simulink model "V2G"  (R2024a)
settings: Solver=ode23tb  StartTime=0.0  StopTime=0.3  MaxStep=1e-6  RelTol=1e-3  EnableMultiTasking=on
undefined symbols (not defined in the file): DiscIntNeverNeededParam, Ion, Lithium
libraries: powerlib_extras x6, spsControlledVoltageSourceLib x5, spsSeriesRLCBranchLib x3, simulink x3, spsCurrentMeasurementLib x3, spsACVoltageSourceLib x3, spsVoltageMeasurementLib x3, spsIGBTDiodeLib x2, dspfdesign x1, spsBatteryLib x1, spsGroundLib x1, spsThreePhaseSeriesRLCBranchLib x1
settings Model: Creator=mengning  LastModifiedBy=徐天明
settings SolverCC: AlgebraicLoopSolver=TrustRegion
settings DataIOCC: LimitDataPoints=on  SaveFormat=Array  ReturnWorkspaceOutputs=off
settings OptimizationCC: LifeSpan=inf
settings DebuggingCC: SolverPrmCheckMsg=warning  UnconnectedInputMsg=warning  UnconnectedOutputMsg=warning  UnconnectedLineMsg=warning  SFUnexpectedBacktrackingDiag=warning  SFNoUnconditionalDefaultTransitionDiag=warning  ArithmeticOperatorsInVariantConditions=warning
settings HardwareCC: ProdBitPerPointer=32  ProdBitPerSizeT=32  ProdBitPerPtrDiffT=32  ProdLargestAtomicFloat=None  ProdIntDivRoundTo=Undefined  ProdEndianess=Unspecified  ProdWordSize=32  ProdHWDeviceType=32-bit Generic
settings ModelReferenceCC: EnableRefExpFcnMdlSchedulingChecks=on  PropagateSignalLabelsOutOfModel=off
settings SFSimCC: SimUseLocalCustomCode=off  CustomCodeUndefinedFunction=UseInterfaceOnly
settings RTWCC: RTWUseLocalCustomCode=off  GPUComputeCapability=3.5
settings CodeAppCC: StateflowObjectComments=on
settings GRTTargetCC: TargetLangStandard=C89/C90 (ANSI)
settings ConfigComp: CovMetricSettings=dw  CovSaveCumulativeToWorkspaceVar=on  CovSaveSingleToWorkspaceVar=on  CovExternalEMLEnable=off  CovSFcnEnable=off
settings SimscapeCC: SimscapeNormalizeSystem=off

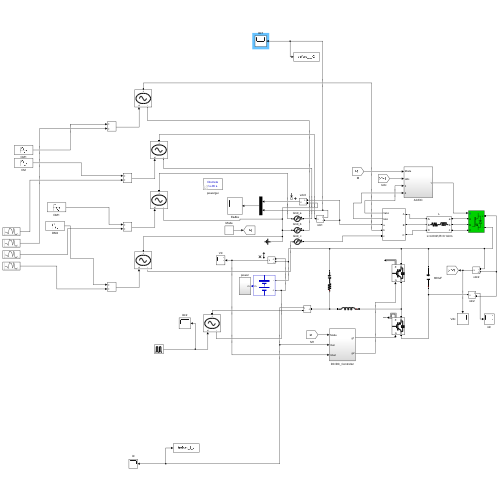
[thumbnail: Simulink's stored preview of the top-level diagram]
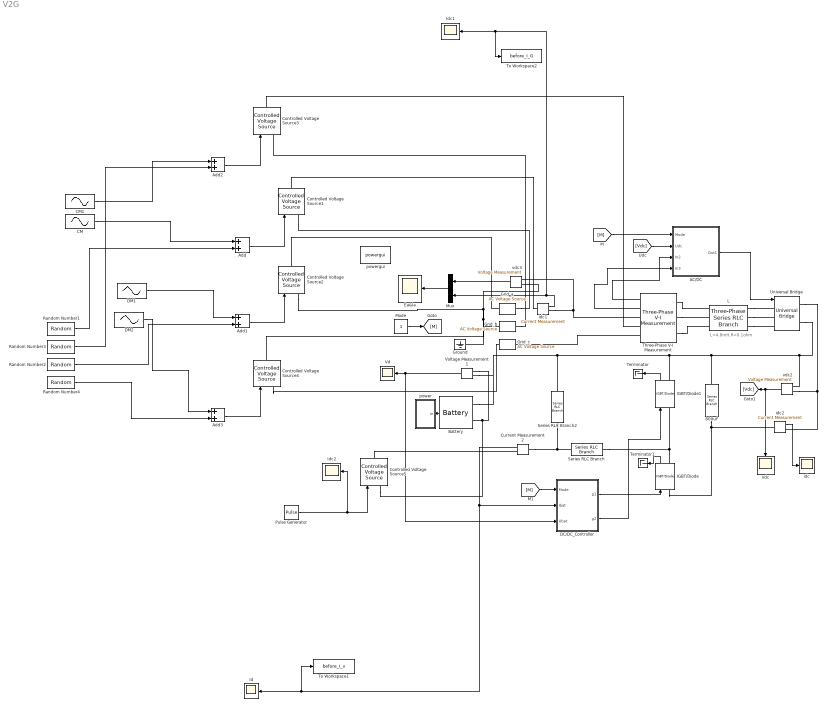
== system V2G ==
  note: L=4.8mH,R=0.1ohm
  800uF : spsSeriesRLCBranchLib/Series RLC Branch  LConnTagsString=__new0  RConnTagsString=__new0  BranchType=C  Resistance=0  Inductance=0  SetiL0=off  InitialCurrent=0  Capacitance=0.0008  Setx0=off  InitialVoltage=0  Measurements=None
  AC/DC : Subsystem
  Add{,1..3} (4 alike) : Sum
  Battery : spsBatteryLib/Battery  BatType=Lithium-Ion  ShowTempParam=off  ThermalPreset=no  ShowAgeParam=off  NomV=200  NomQ=96  SOC=90  Batt_Tr=0.001  PresetModel=off  MaxQ=100  MinV=150  FullV=350  Dis_rate=50  R=0.04  Normal_OP=48.0769  expZone="[216.9492            10]"  current=[1.5 3]  Units=Ampere-hour  Tci=20  NomT=25  T2=0  MaxQ2=2.208  FullV2=3.45  Normal_OP2=2.8  expZone2="[3.22        0.23]"  Rca=0.6  ti=1000  Dp=0  Neq0=0  Tsim=1e6  Ta1=25  Qeol=5.4*0.9  Reol=0.013333*1.2  Char_age=[2.3478, 3]  Dis_age=[2.3478, 10]  N1=1500  N2=10500  N3=1000  N4=1400  Ta2=45  N5=950
      settings: LibrarySourceBlock=electricdrivelib/Extra Sources/Battery
  CM : Sin  Amplitude=3  Frequency=500  SampleTime=0
  CM1 : Sin  Amplitude=3  Frequency=500  SampleTime=0
  Controlled Voltage Source{1..5} (5 alike) : spsControlledVoltageSourceLib/Controlled Voltage Source  Initialize=on  Source_Type=AC  Amplitude=0  Phase=0  Frequency=0  Measurements=None
  Current Measurement2 : spsCurrentMeasurementLib/Current Measurement  PhasorSimulation=off  OutputType=Complex  PSBequivalent=0
  DC/DC_Controller : Subsystem
  DM1 : Sin  Amplitude=30  Frequency=50  SampleTime=0
  DM2 : Sin  Amplitude=30  Frequency=50  SampleTime=0
  Ea&Ia : Scope
  Grid_a : spsACVoltageSourceLib/AC Voltage Source  Amplitude=311  Phase=90  Frequency=50  SampleTime=0  Measurements=None  BusType=swing  Pref=10e3  Qref=0  Qmin=-inf  Qmax=+inf
  Grid_b : spsACVoltageSourceLib/AC Voltage Source  Amplitude=311  Phase=-120+90  Frequency=50  SampleTime=0  Measurements=None  BusType=swing  Pref=10e3  Qref=0  Qmin=-inf  Qmax=+inf
  Grid_c : spsACVoltageSourceLib/AC Voltage Source  Amplitude=311  Phase=-240+90  Frequency=50  SampleTime=0  Measurements=None  BusType=swing  Pref=10e3  Qref=0  Qmin=-inf  Qmax=+inf
  Ground : spsGroundLib/Ground  LConnTagsString=a
  IGBT/Diode : spsIGBTDiodeLib/IGBT//Diode  Ron=1e-3  Rs=1e5  Cs=inf  Measurements=on
  IGBT/Diode1 : spsIGBTDiodeLib/IGBT//Diode  Ron=1e-3  Rs=1e5  Cs=inf  Measurements=on
  Id : Scope
  Idc1 : Scope
  Idc2 : Scope
  L : spsThreePhaseSeriesRLCBranchLib/Three-Phase Series RLC Branch  LConnTagsString=A|B|C  RConnTagsString=A|B|C  BranchType=RL  Resistance=0.1  Inductance=17e-3  Capacitance=1.0  Measurements=None
  Mode : Constant
  Mux : Mux  Inputs=2
  Pulse Generator : DiscretePulseGenerator  PulseType=Time based  Amplitude=1000  Period=10  PulseWidth=99  PhaseDelay=0.05
  Random Number1 : RandomNumber  Mean=60  Variance=20  SampleTime=0
  Random Number2 : RandomNumber  Variance=10  SampleTime=0
  Random Number3 : RandomNumber  Variance=20  SampleTime=0
  Random Number4 : RandomNumber  Variance=10  SampleTime=0
  Series RLC Branch : spsSeriesRLCBranchLib/Series RLC Branch  LConnTagsString=__new0  RConnTagsString=__new0  BranchType=L  Resistance=0.1  Inductance=0.032  SetiL0=on  InitialCurrent=5  Capacitance=1e-6  Setx0=off  InitialVoltage=0  Measurements=None
  Series RLC Branch2 : spsSeriesRLCBranchLib/Series RLC Branch  LConnTagsString=__new0  RConnTagsString=__new0  BranchType=RC  Resistance=0.15  Inductance=5e-3  SetiL0=off  InitialCurrent=0  Capacitance=0.00033  Setx0=on  InitialVoltage=220  Measurements=None
  Terminator : Terminator
  Terminator1 : Terminator
  Three-Phase V-I Measurement : spsThreePhaseVIMeasurementLib/Three-Phase V-I Measurement  VoltageMeasurement=phase-to-ground  SetLabelV=off  LabelV=Vabc  Vpu=off  VpuLL=off  CurrentMeasurement=yes  SetLabelI=off  LabelI=Iabc  Ipu=off  Pbase=100e6  Vbase=500e3  OutputType=Complex  PhasorSimulation=off  PSBequivalent=0
  To Workspace1 : ToWorkspace  VariableName=before_I_v  SaveFormat=Timeseries  SampleTime=-1
  To Workspace2 : ToWorkspace  VariableName=before_I_G  SaveFormat=Timeseries  SampleTime=-1
  Universal Bridge : spsUniversalBridgeLib/Universal Bridge  Arms=3  SnubberResistance=1e5  SnubberCapacitance=inf  Device=IGBT / Diodes  Ron=1e-3  Lon=0  ForwardVoltages="[  0  0  ]"  ForwardVoltage=0  GTOparameters=[ 10e-6 , 20e-6 ]  IGBTparameters=[ 1e-6 , 2e-6 ]  Measurements=None  Measurements_2=None  converterType=Rectifier
  Vd : Scope
  Vdc : Scope
  Voltage Measurement1 : spsVoltageMeasurementLib/Voltage Measurement  PhasorSimulation=off  OutputType=Complex  PSBequivalent=0
  idc : Scope
  idc1 : spsCurrentMeasurementLib/Current Measurement  PhasorSimulation=off  OutputType=Complex  PSBequivalent=0
  idc2 : spsCurrentMeasurementLib/Current Measurement  PhasorSimulation=off  OutputType=Complex  PSBequivalent=0
  power : Subsystem
  powergui : sps_lib/powergui  Priority=1  SimulationMode=Discrete  SampleTime=1e-6  frequency=60  Iterations=50  frequencyindice=0  Pbase=100e6  ErrMax=1e-4  UnitsV=kV  UnitsW=MW  buscounter=0  FunctionMessages=off  echomessages=off  EnableUseOfTLC=off  CurrentSourceSwitches=off  DisableSnubberDevices=off  DisableRonSwitches=off  DisableVfSwitches=off  DisplayEquations=off  AutomaticDiscreteSolvers=off  SolverType=Tustin  Interpol=off  ExternalGateDelay=off  methode=off  Ts=0  x0status=blocks  SPID=off  SwTol=0  HookPort=off  NonlinearTolerance=1e-4  nMaxIteration=100  ContinueOnMaxIteration=off  RestoreLinks=warning  ResistiveCurrentMeasurement=off  Frange=[0:2:500]  Ylog=off  Xlog=on  ShowGrid=off  save=off  variable=ZData  structure=ScopeData  ZoomFFT=off  StartTime=0.0  cycles=1  DisplayStyle=1  fundamental=60  FreqAxis=off  MaxFrequency=1000  frequencyindicesteady=1  RmsSteady=1  display=off
  vdc2 : spsVoltageMeasurementLib/Voltage Measurement  PhasorSimulation=off  OutputType=Complex  PSBequivalent=0
  vdc3 : spsVoltageMeasurementLib/Voltage Measurement  PhasorSimulation=off  OutputType=Complex  PSBequivalent=0
  wires:
  Mux/1 -> Ea&Ia/1
  vdc3/1 -> Mux/1
  idc1/1 -> To Workspace2/1, Idc1/1, Mux/2
  Three-Phase V-I Measurement/1 -> AC/DC/3(In2)
  Three-Phase V-I Measurement/2 -> AC/DC/4(In3)
  AC/DC/1(Out1) -> Universal Bridge/1
  [Vdc] -> AC/DC/2(Udc)
  Mode/1 -> [M]
  [M] -> AC/DC/1(Mode)
  DC/DC_Controller/1(g1) -> IGBT/Diode/1
  DC/DC_Controller/2(g2) -> IGBT/Diode1/1
  Battery/1 -> power/1(m)
  vdc2/1 -> [Vdc], Vdc/1
  idc2/1 -> idc/1
  IGBT/Diode1/1 -> Terminator/1
  IGBT/Diode/1 -> Terminator1/1
  [M] -> DC/DC_Controller/1(Mode)
  Voltage Measurement1/1 -> DC/DC_Controller/3(Ubat), Vd/1
  Current Measurement2/1 -> DC/DC_Controller/2(Ibat), To Workspace1/1, Id/1
  Add/1 -> Controlled Voltage Source1/1
  Random Number1/1 -> Add/2
  Add1/1 -> Controlled Voltage Source2/1
  DM1/1 -> Add1/1
  Random Number2/1 -> Add1/2
  CM/1 -> Add/1
  Add2/1 -> Controlled Voltage Source3/1
  CM1/1 -> Add2/1
  Random Number4/1 -> Add3/2
  Add3/1 -> Controlled Voltage Source4/1
  DM2/1 -> Add3/1
  Random Number3/1 -> Add2/2
  Pulse Generator/1 -> Controlled Voltage Source5/1, Idc2/1
  connections:
  Controlled Voltage Source4/RConn1 -- Ground/LConn1 -- Grid_b/LConn1 -- Controlled Voltage Source2/LConn1 -- vdc3/LConn2
  Three-Phase V-I Measurement/RConn1 -- idc1/RConn1 -- vdc3/LConn1
  Three-Phase V-I Measurement/LConn3 -- L/LConn3
  L/RConn1 -- Universal Bridge/LConn1
  L/RConn3 -- Universal Bridge/LConn3
  Three-Phase V-I Measurement/LConn2 -- L/LConn2
  L/RConn2 -- Universal Bridge/LConn2
  Three-Phase V-I Measurement/LConn1 -- L/LConn1
  Universal Bridge/RConn1 -- vdc2/LConn1 -- idc2/RConn1
  800uF/LConn1 -- IGBT/Diode/LConn1 -- idc2/LConn1
  Universal Bridge/RConn2 -- vdc2/LConn2 -- Battery/LConn2 -- Voltage Measurement1/LConn2 -- Series RLC Branch2/RConn1 -- IGBT/Diode1/RConn1 -- 800uF/RConn1
  IGBT/Diode/RConn1 -- Series RLC Branch/LConn1 -- IGBT/Diode1/LConn1
  Series RLC Branch2/LConn1 -- Series RLC Branch/RConn1 -- Current Measurement2/LConn1
  Voltage Measurement1/LConn1 -- Controlled Voltage Source5/LConn1 -- Battery/LConn1
  Grid_a/RConn1 -- Controlled Voltage Source1/LConn1
  Controlled Voltage Source1/RConn1 -- idc1/LConn1
  Grid_b/RConn1 -- Controlled Voltage Source3/LConn1
  Controlled Voltage Source3/RConn1 -- Three-Phase V-I Measurement/RConn2
  Grid_a/LConn1 -- Controlled Voltage Source2/RConn1
  Controlled Voltage Source4/LConn1 -- Grid_c/LConn1
  Grid_c/RConn1 -- Three-Phase V-I Measurement/RConn3
  Controlled Voltage Source5/RConn1 -- Current Measurement2/RConn1

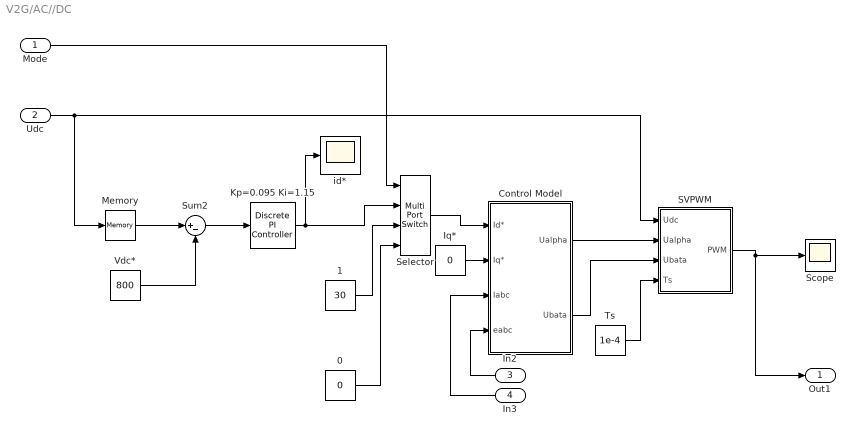
== system V2G/AC//DC ==
  Mode : Inport
  Udc : Inport  Port=2
  In2 : Inport  Port=3
  In3 : Inport  Port=4
  0 : Constant  Value=0
  1 : Constant  Value=30
  Control Model : Subsystem
  Iq* : Constant  Value=0
  Kp=0.095 Ki=1.15 : powerlib_extras/Discrete  Control Blocks/Discrete PI Controller  Kp=0.095  Ki=1.15  Par_Limits=[10e6 -10e6]  Init=0  Ts=50e-6
  Memory : Memory  InitialCondition=1e-5
  "SVPWM " : Subsystem
  Scope : Scope
  Selector : MultiPortSwitch  DiagnosticForDefault=None  SaturateOnIntegerOverflow=off  InputSameDT=off
  Sum2 : Sum  Inputs=|+-
  Ts : Constant  Value=1e-4
  Vdc* : Constant  Value=800
  id* : Scope
  Out1 : Outport
  wires:
  Vdc*/1 -> Sum2/2
  Sum2/1 -> Kp=0.095 Ki=1.15/1
  Iq*/1 -> Control Model/2(Iq*)
  In2/1 -> Control Model/4(eabc)
  In3/1 -> Control Model/3(Iabc)
  Control Model/2(Ubata) -> "SVPWM "/3(Ubata)
  Ts/1 -> "SVPWM "/4(Ts)
  Memory/1 -> Sum2/1
  Udc/1 -> Memory/1, "SVPWM "/1(Udc)
  "SVPWM "/1(PWM) -> Out1/1, Scope/1
  Kp=0.095 Ki=1.15/1 -> id*/1, Selector/2
  Control Model/1(Ualpha) -> "SVPWM "/2(Ualpha)
  Mode/1 -> Selector/1
  0/1 -> Selector/4
  1/1 -> Selector/3
  Selector/1 -> Control Model/1(Id*)

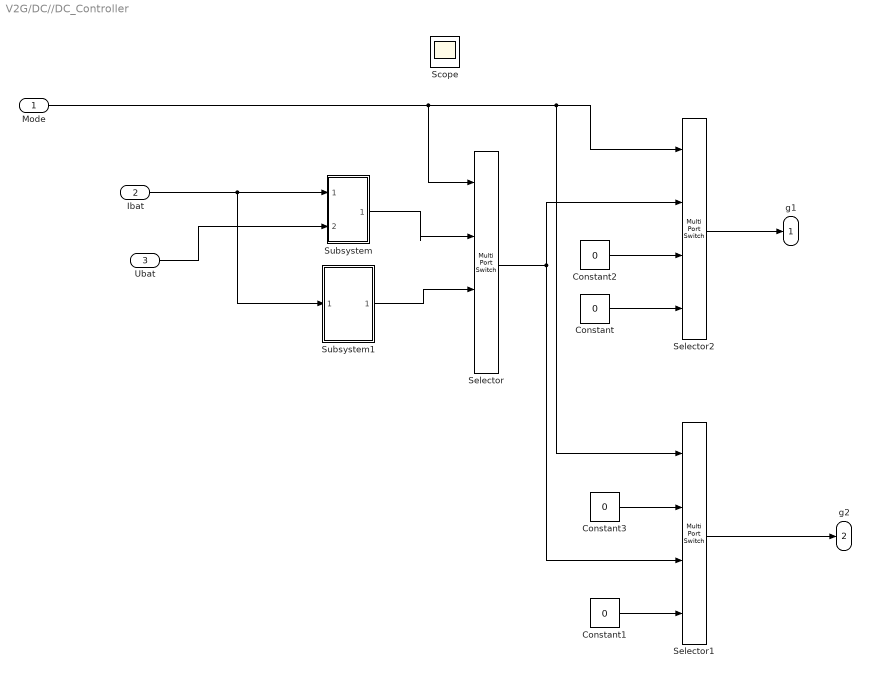
== system V2G/DC//DC_Controller ==
  Mode : Inport
  Ibat : Inport  Port=2
  Ubat : Inport  Port=3
  Constant{,1..3} (4 alike) : Constant  Value=0
  Scope : Scope
  Selector : MultiPortSwitch  DiagnosticForDefault=None  SaturateOnIntegerOverflow=off  InputSameDT=off
  Selector1 : MultiPortSwitch  DiagnosticForDefault=None  SaturateOnIntegerOverflow=off  InputSameDT=off
  Selector2 : MultiPortSwitch  DiagnosticForDefault=None  SaturateOnIntegerOverflow=off  InputSameDT=off
  Subsystem : Subsystem
  Subsystem1 : Subsystem
  g1 : Outport
  g2 : Outport  Port=2
  wires:
  Ubat/1 -> Subsystem/2(Ubat)
  Ibat/1 -> Subsystem1/1(Ibat2), Subsystem/1(Ibat)
  Subsystem/1(Out1) -> Selector/2
  Subsystem1/1(out2) -> Selector/3
  Selector/1 -> Selector2/2, Selector1/3
  Constant/1 -> Selector2/4
  Constant1/1 -> Selector1/4
  Constant2/1 -> Selector2/3
  Constant3/1 -> Selector1/2
  Mode/1 -> Selector/1, Selector1/1, Selector2/1
  Selector2/1 -> g1/1
  Selector1/1 -> g2/1

== system V2G/power ==
  m : Inport
  Demux1 : Demux  Outputs=3
  Scope : Scope
  Scope1 : Scope
  Scope10 : Scope
  Terminator : Terminator
  To Workspace : ToWorkspace  VariableName=Ibat1  SampleTime=1e-6
  wires:
  Demux1/3 -> Terminator/1, Scope1/1
  m/1 -> Demux1/1
  Demux1/1 -> Scope/1, [SOC]
  Demux1/2 -> Scope10/1, To Workspace/1, [I_bat]

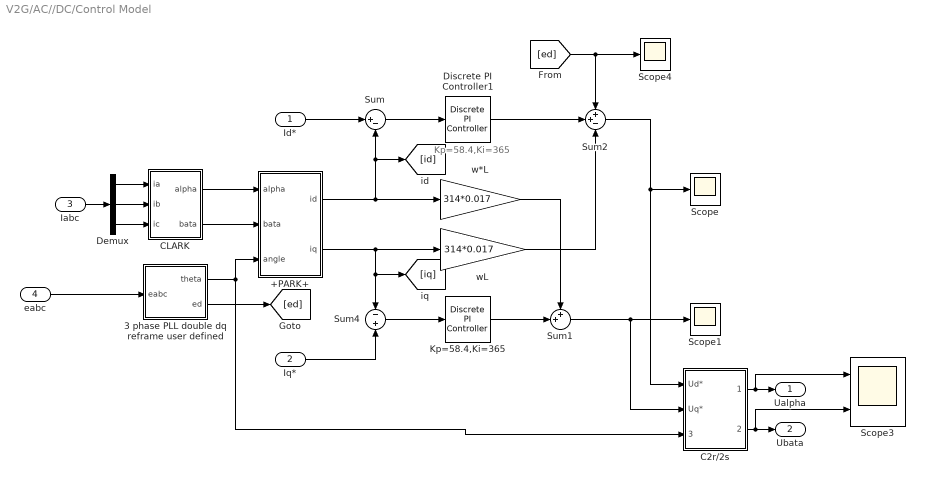
== system V2G/AC//DC/Control Model ==
  note: Kp=58.4,Ki=365
  Id* : Inport
  Iq* : Inport  Port=2
  Iabc : Inport  Port=3
  eabc : Inport  Port=4
  +PARK+ : Subsystem
  3 phase PLL double dq reframe user defined : Subsystem
  C2r/2s : Subsystem
  CLARK : Subsystem
  Demux : Demux  Outputs=3
  Discrete PI Controller1 : powerlib_extras/Discrete  Control Blocks/Discrete PI Controller  Kp=58.4  Ki=365  Par_Limits=[10e6 -10e6]  Init=0  Ts=50e-6
  Kp=58.4,Ki=365 : powerlib_extras/Discrete  Control Blocks/Discrete PI Controller  Kp=58.4  Ki=365  Par_Limits=[10e6 -10e6]  Init=0  Ts=50e-6
  Scope : Scope
  Scope1 : Scope
  Scope3 : Scope  NumInputPorts=2
  Scope4 : Scope
  Sum : Sum  Inputs=|+-
  Sum1 : Sum  Inputs=++|
  Sum2 : Sum  Inputs=++-
  Sum4 : Sum  Inputs=-+
  w*L : Gain  Gain=314*0.017
  wL : Gain  Gain=314*0.017
  Ualpha : Outport
  Ubata : Outport  Port=2
  wires:
  Iabc/1 -> Demux/1
  Demux/1 -> CLARK/1(ia)
  Demux/2 -> CLARK/2(ib)
  Demux/3 -> CLARK/3(ic)
  CLARK/2(bata) -> +PARK+/2(bata)
  CLARK/1(alpha) -> +PARK+/1(alpha)
  Id*/1 -> Sum/1
  +PARK+/1(id) -> w*L/1, Sum/2, [id]
  Iq*/1 -> Sum4/2
  +PARK+/2(iq) -> wL/1, Sum4/1, [iq]
  Sum4/1 -> Kp=58.4,Ki=365/1
  Sum/1 -> Discrete PI Controller1/1
  C2r/2s/1(Ualpha) -> Ualpha/1, Scope3/1
  Sum1/1 -> C2r/2s/2(Uq*), Scope1/1
  C2r/2s/2(Ubata) -> Ubata/1, Scope3/2
  Sum2/1 -> C2r/2s/1(Ud*), Scope/1
  [ed] -> Scope4/1, Sum2/1
  Kp=58.4,Ki=365/1 -> Sum1/2
  w*L/1 -> Sum1/1
  Discrete PI Controller1/1 -> Sum2/2
  wL/1 -> Sum2/3
  eabc/1 -> 3 phase PLL double dq reframe user defined/1(eabc)
  3 phase PLL double dq reframe user defined/1(theta) -> +PARK+/3(angle), C2r/2s/3(angle)
  3 phase PLL double dq reframe user defined/2(ed) -> [ed]

== system V2G/AC//DC/SVPWM  ==
  Udc : Inport
  Ualpha : Inport  Port=2
  Ubata : Inport  Port=3
  Ts : Inport  Port=4
  " " : Subsystem
  Memory{,1..3} (4 alike) : Memory  InitialCondition=5e-6
  Mux : Mux  Inputs=6
  PWM Generation : Subsystem
  XYZ : Subsystem
  Zone : Subsystem
  switch time : Subsystem
  PWM : Outport
  wires:
  Mux/1 -> PWM/1
  PWM Generation/5(PWM5) -> Mux/5
  switch time/3(" Tcm3") -> PWM Generation/3(Tcm3)
  switch time/2(" Tcm2") -> PWM Generation/2(Tcm2)
  switch time/1(Tcm1) -> PWM Generation/1(Tcm1)
  " "/2(Ty) -> switch time/3(Ty)
  " "/1(Tx) -> switch time/2(Tx)
  PWM Generation/6(PWM6) -> Mux/6
  PWM Generation/4(PWM4) -> Mux/4
  PWM Generation/3(PWM3) -> Mux/3
  PWM Generation/2(PWM2) -> Mux/2
  PWM Generation/1(PWM1) -> Mux/1
  Udc/1 -> Memory3/1
  Ts/1 -> Memory2/1
  XYZ/3(Z) -> " "/4(Z)
  XYZ/2(Y) -> " "/3(Y)
  XYZ/1(X) -> " "/2(X)
  Zone/1(n) -> switch time/1(n), " "/1(n)
  Ubata/1 -> Memory1/1
  Ualpha/1 -> Memory/1
  Memory/1 -> Zone/1(Ualph), XYZ/1(Ualph)
  Memory1/1 -> Zone/2(Ubata), XYZ/2(Ubata)
  Memory2/1 -> " "/5(Ts), switch time/4(Ts), XYZ/3(T)
  Memory3/1 -> XYZ/4(Udc)

== system V2G/DC//DC_Controller/Subsystem ==
  Ibat : Inport
  Ubat : Inport  Port=2
  " " : powerlib_extras/Discrete  Control Blocks/Discrete PI Controller  Kp=4.75  Ki=24.67  Par_Limits=[10e6 -10e6]  Init=0  Ts=50e-6
  " " : powerlib_extras/Discrete  Control Blocks/Discrete PI Controller  Kp=24  Ki=1.3  Par_Limits=[10e6 -10e6]  Init=0  Ts=50e-6
  Idc1 : Scope
  "PWM " : Subsystem
  Saturation1 : Saturate  UpperLimit=1  LowerLimit=0
  Saturation2 : Saturate  UpperLimit=20  LowerLimit=0
  Scope : Scope
  Scope1 : Scope
  Sum3 : Sum  Inputs=|+-
  Sum4 : Sum  Inputs=+-
  Uref : Constant  Value=230
  Out1 : Outport
  wires:
  Ubat/1 -> Sum3/2
  Ibat/1 -> Sum4/2
  Saturation1/1 -> Scope1/1, "PWM "/1(D)
  Sum3/1 -> " "/1
  " "/1 -> Saturation2/1
  Sum4/1 -> " "/1
  " "/1 -> Scope/1, Saturation1/1
  Uref/1 -> Sum3/1
  Saturation2/1 -> Idc1/1, Sum4/1
  "PWM "/1(PWM) -> Out1/1

== system V2G/DC//DC_Controller/Subsystem1 ==
  Ibat2 : Inport
  Discrete PI Controller2 : Subsystem  AncestorBlock=|  mask(Discrete PI Controller){Kp=1.2, Ki=80, Par_Limits=[5000 -5000], Init=0, Ts=1e-4}
      | powerlib_extras/Discrete 
      | Control Blocks/Discrete
      | PI Controller
      mask prompts: Kp "Proportional gain (Kp):"; Ki "Integral gain (Ki):"; Par_Limits "Output limits: [ Upper   Lower ]"; Init "Output initial value:"; Ts "Sample time:"
      mask help: This block implements a discrete PI controller.
      mask init:
      | UpperLimit=Par_Limits(1);
      | LowerLimit=Par_Limits(2);
      mask Display: disp('PI');
  Gain : Gain  Gain=-1
  Iref2 : Constant  Value=34
  "PWM " : Subsystem
  Saturation2 : Saturate  UpperLimit=1  LowerLimit=0
  Sum : Sum  Inputs=|+-
  out2 : Outport
  wires:
  Sum/1 -> Discrete PI Controller2/1(Error)
  Discrete PI Controller2/1(Out) -> Saturation2/1
  Saturation2/1 -> "PWM "/1(D)
  "PWM "/1(PWM) -> out2/1
  Gain/1 -> Sum/1
  Iref2/1 -> Gain/1
  Ibat2/1 -> Sum/2

== system V2G/AC//DC/Control Model/+PARK+ ==
  alpha : Inport
  bata : Inport  Port=2
  angle : Inport  Port=3
  Fcn : Fcn  Expr=u(1)*cos(u(3))+u(2)*sin(u(3))
  Fcn1 : Fcn  Expr=-u(1)*sin(u(3))+u(2)*cos(u(3))
  Mux : Mux  Inputs=3
  Scope1 : Scope  NumInputPorts=2
  id : Outport
  iq : Outport  Port=2
  wires:
  alpha/1 -> Mux/1
  bata/1 -> Mux/2
  angle/1 -> Mux/3
  Mux/1 -> Fcn/1, Fcn1/1
  Fcn1/1 -> Scope1/2, iq/1
  Fcn/1 -> id/1, Scope1/1

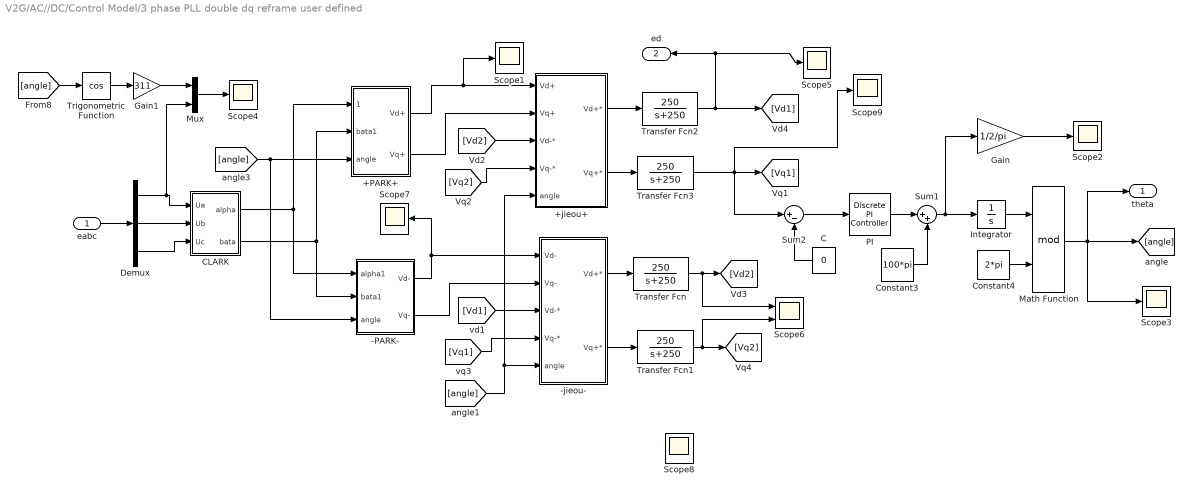
== system V2G/AC//DC/Control Model/3 phase PLL double dq reframe user defined ==
  eabc : Inport
  +PARK+ : Subsystem
  +jieou+ : Subsystem
  -PARK- : Subsystem
  -jieou- : Subsystem
  C : Constant  Value=0
  CLARK : Subsystem
  Constant3 : Constant  Value=100*pi
  Constant4 : Constant  Value=2*pi
  Demux : Demux  Outputs=3
  Gain : Gain  Gain=1/2/pi
  Gain1 : Gain  Gain=311
  Integrator : Integrator
  Math Function : Math  Operator=mod  SignedPower=on
  Mux : Mux  Inputs=2
  PI : powerlib_extras/Discrete  Control Blocks/Discrete PI Controller  Kp=150  Ki=1000  Par_Limits=[1e6 -1e6]  Init=0  Ts=50e-6
  Scope{1..5,7..9} (8 alike) : Scope
  Scope6 : Scope  NumInputPorts=2
  Sum1 : Sum  Inputs=|++
  Sum2 : Sum  Inputs=|+-
  Transfer Fcn{,1..3} (4 alike) : TransferFcn  Numerator=[250]  Denominator=[1 250]
  Trigonometric Function : Trigonometry  Operator=cos
  theta : Outport
  ed : Outport  Port=2
  wires:
  CLARK/1(alpha) -> +PARK+/1(alpha1), -PARK-/1(alpha1)
  CLARK/2(bata) -> +PARK+/2(bata1), -PARK-/2(bata1)
  [angle] -> +PARK+/3(angle), -PARK-/3(angle)
  +PARK+/1(Vd+) -> +jieou+/1(Vd+), Scope1/1
  +PARK+/2(Vq+) -> +jieou+/2(Vq+)
  +jieou+/1(Vd+*) -> Transfer Fcn2/1
  +jieou+/2(Vq+*) -> Transfer Fcn3/1
  Transfer Fcn2/1 -> [Vd1], Scope5/1, ed/1
  Transfer Fcn3/1 -> Scope9/1, Sum2/1, [Vq1]
  Transfer Fcn/1 -> [Vd2], Scope6/1
  Transfer Fcn1/1 -> [Vq2], Scope6/2
  [Vd2] -> +jieou+/3(Vd-*)
  [Vq2] -> +jieou+/4(Vq-*)
  PI/1 -> Sum1/1
  Constant3/1 -> Sum1/2
  Sum1/1 -> Integrator/1, Gain/1
  Integrator/1 -> Math Function/1
  Constant4/1 -> Math Function/2
  Gain/1 -> Scope2/1
  Math Function/1 -> [angle], Scope3/1, theta/1
  [angle] -> Trigonometric Function/1
  Trigonometric Function/1 -> Gain1/1
  eabc/1 -> Demux/1
  Demux/1 -> Mux/2, CLARK/1(Ua)
  Demux/2 -> CLARK/2(Ub)
  Demux/3 -> CLARK/3(Uc)
  [angle] -> +jieou+/5(angle), -jieou-/5(angle)
  Sum2/1 -> PI/1
  C/1 -> Sum2/2
  -PARK-/1(Vd-) -> -jieou-/1(Vd-), Scope7/1
  -PARK-/2(Vq-) -> -jieou-/2(Vq-)
  [Vd1] -> -jieou-/3(Vd-*)
  [Vq1] -> -jieou-/4(Vq-*)
  -jieou-/1(Vd+*) -> Transfer Fcn/1
  -jieou-/2(Vq+*) -> Transfer Fcn1/1
  Mux/1 -> Scope4/1
  Gain1/1 -> Mux/1

== system V2G/AC//DC/Control Model/C2r//2s ==
  Ud* : Inport
  Uq* : Inport  Port=2
  angle : Inport  Port=3
  Fcn : Fcn  Expr=u(1)*cos(u(3))-u(2)*sin(u(3))
  Fcn1 : Fcn  Expr=u(1)*sin(u(3))+u(2)*cos(u(3))
  Mux : Mux  Inputs=3
  Scope : Scope  NumInputPorts=2
  Ualpha : Outport
  Ubata : Outport  Port=2
  wires:
  Ud*/1 -> Mux/1
  Uq*/1 -> Mux/2
  Mux/1 -> Fcn/1, Fcn1/1
  Fcn1/1 -> Ubata/1, Scope/2
  Fcn/1 -> Ualpha/1, Scope/1
  angle/1 -> Mux/3

== system V2G/AC//DC/Control Model/CLARK ==
  ia : Inport
  ib : Inport  Port=2
  ic : Inport  Port=3
  Fcn : Fcn  Expr=(2*u(1)-u(2)-u(3))/3
  Fcn1 : Fcn  Expr=(u(2)-u(3))*sqrt(3)/3
  Mux : Mux  Inputs=3
  Scope : Scope  NumInputPorts=2
  alpha : Outport
  bata : Outport  Port=2
  wires:
  ia/1 -> Mux/1
  ib/1 -> Mux/2
  ic/1 -> Mux/3
  Mux/1 -> Fcn/1, Fcn1/1
  Fcn/1 -> alpha/1, Scope/1
  Fcn1/1 -> bata/1, Scope/2

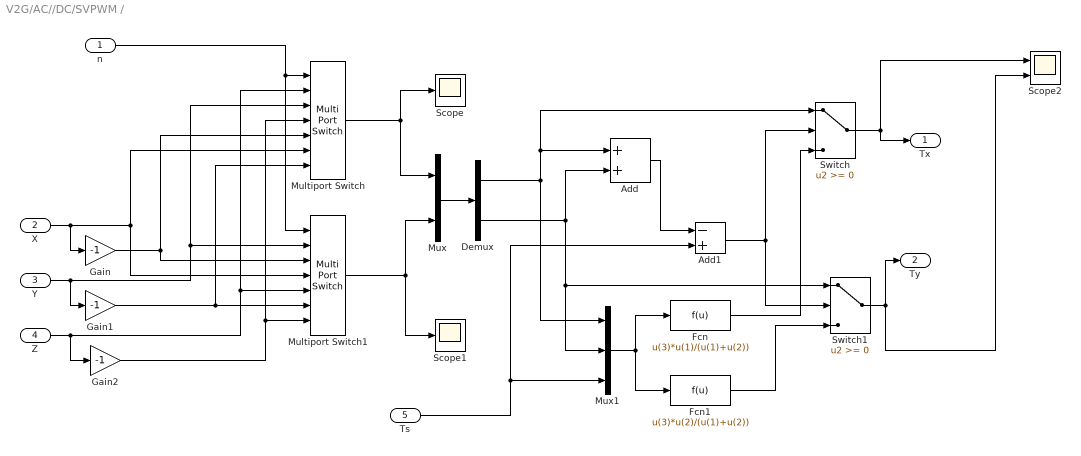
== system V2G/AC//DC/SVPWM /  ==
  n : Inport
  X : Inport  Port=2
  Y : Inport  Port=3
  Z : Inport  Port=4
  Ts : Inport  Port=5
  Add : Sum
  Add1 : Sum  Inputs=-+
  Demux : Demux  Outputs=2
  Fcn : Fcn  Expr=u(3)*u(1)/(u(1)+u(2))
  Fcn1 : Fcn  Expr=u(3)*u(2)/(u(1)+u(2))
  Gain : Gain  Gain=-1
  Gain1 : Gain  Gain=-1
  Gain2 : Gain  Gain=-1
  Multiport Switch : MultiPortSwitch  Inputs=6  SaturateOnIntegerOverflow=off  InputSameDT=off
  Multiport Switch1 : MultiPortSwitch  Inputs=6  SaturateOnIntegerOverflow=off  InputSameDT=off
  Mux : Mux  Inputs=2
  Mux1 : Mux  Inputs=3
  Scope : Scope
  Scope1 : Scope
  Scope2 : Scope  NumInputPorts=2
  Switch : Switch  SaturateOnIntegerOverflow=off  InputSameDT=off
  Switch1 : Switch  SaturateOnIntegerOverflow=off  InputSameDT=off
  Tx : Outport
  Ty : Outport  Port=2
  wires:
  Mux/1 -> Demux/1
  Switch1/1 -> Scope2/2, Ty/1
  Demux/1 -> Add/1, Switch/1, Mux1/1
  Switch/1 -> Tx/1, Scope2/1
  Multiport Switch/1 -> Mux/1, Scope/1
  Multiport Switch1/1 -> Mux/2, Scope1/1
  Fcn1/1 -> Switch1/3
  Fcn/1 -> Switch/3
  Mux1/1 -> Fcn1/1, Fcn/1
  Add1/1 -> Switch1/2, Switch/2
  Add/1 -> Add1/1
  Ts/1 -> Mux1/3, Add1/2
  Demux/2 -> Switch1/1, Mux1/2, Add/2
  n/1 -> Multiport Switch1/1, Multiport Switch/1
  Gain/1 -> Multiport Switch1/3, Multiport Switch/5
  Gain1/1 -> Multiport Switch/7, Multiport Switch1/6
  Gain2/1 -> Multiport Switch1/7, Multiport Switch/4
  Z/1 -> Gain2/1, Multiport Switch/2, Multiport Switch1/5
  Y/1 -> Gain1/1, Multiport Switch1/2, Multiport Switch/3
  X/1 -> Gain/1, Multiport Switch/6, Multiport Switch1/4

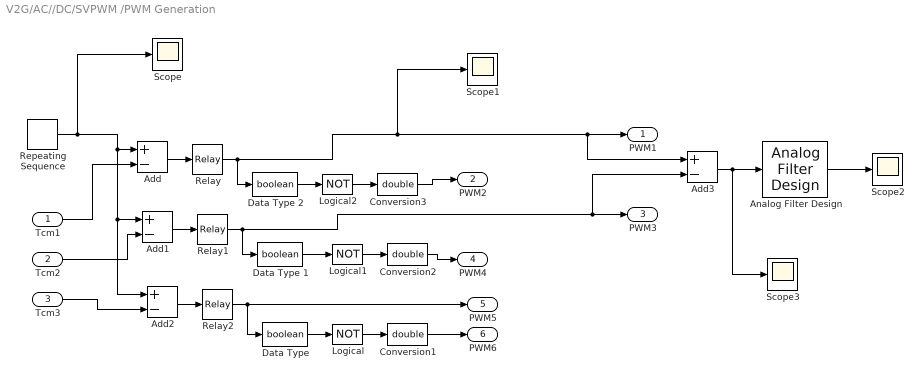
== system V2G/AC//DC/SVPWM /PWM Generation ==
  Tcm1 : Inport
  Tcm2 : Inport  Port=2
  Tcm3 : Inport  Port=3
  " Conversion1" : DataTypeConversion  OutDataTypeStr=double  SaturateOnIntegerOverflow=off  RndMeth=Floor
  " Conversion3" : DataTypeConversion  OutDataTypeStr=double  SaturateOnIntegerOverflow=off  RndMeth=Floor
  Add{,1..3} (4 alike) : Sum  Inputs=+-
  Analog Filter Design : dspfdesign/Analog Filter Design  method=Butterworth  filttype=Lowpass  N=8  Wlo=100*pi  Whi=80  Rp=2  Rs=40
  Conversion2 : DataTypeConversion  OutDataTypeStr=double  SaturateOnIntegerOverflow=off  RndMeth=Floor
  "Data Type " : DataTypeConversion  OutDataTypeStr=boolean  SaturateOnIntegerOverflow=off  RndMeth=Floor
  Data Type 1 : DataTypeConversion  OutDataTypeStr=boolean  SaturateOnIntegerOverflow=off  RndMeth=Floor
  Data Type 2 : DataTypeConversion  OutDataTypeStr=boolean  SaturateOnIntegerOverflow=off  RndMeth=Floor
  "Logical " : Logic  Operator=NOT  AllPortsSameDT=off  OutDataTypeStr=boolean
  Logical1 : Logic  Operator=NOT  AllPortsSameDT=off  OutDataTypeStr=boolean
  Logical2 : Logic  Operator=NOT  AllPortsSameDT=off  OutDataTypeStr=boolean
  Relay : Relay
  Relay1 : Relay
  Relay2 : Relay
  Repeating Sequence : simulink/Sources/Repeating Sequence  rep_seq_t=[0 0.5e-4 1e-4]  rep_seq_y=[0 0.5e-4 0]
  Scope{,1..3} (4 alike) : Scope
  PWM1 : Outport
  PWM2 : Outport  Port=2
  PWM3 : Outport  Port=3
  PWM4 : Outport  Port=4
  PWM5 : Outport  Port=5
  PWM6 : Outport  Port=6
  wires:
  Analog Filter Design/1 -> Scope2/1
  Add3/1 -> Scope3/1, Analog Filter Design/1
  " Conversion1"/1 -> PWM6/1
  "Logical "/1 -> " Conversion1"/1
  "Data Type "/1 -> "Logical "/1
  Relay1/1 -> Add3/2, PWM3/1, Data Type 1/1
  Conversion2/1 -> PWM4/1
  Logical1/1 -> Conversion2/1
  Data Type 1/1 -> Logical1/1
  Logical2/1 -> " Conversion3"/1
  Data Type 2/1 -> Logical2/1
  " Conversion3"/1 -> PWM2/1
  Relay/1 -> Add3/1, PWM1/1, Scope1/1, Data Type 2/1
  Relay2/1 -> "Data Type "/1, PWM5/1
  Add2/1 -> Relay2/1
  Add1/1 -> Relay1/1
  Add/1 -> Relay/1
  Tcm3/1 -> Add2/2
  Tcm2/1 -> Add1/2
  Repeating Sequence/1 -> Scope/1, Add/1, Add1/1, Add2/1
  Tcm1/1 -> Add/2

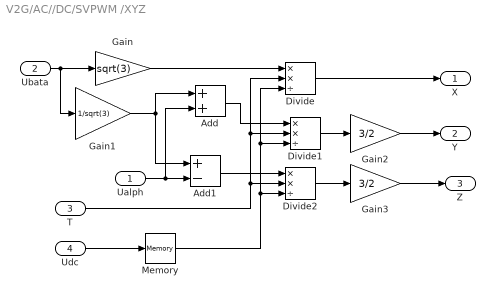
== system V2G/AC//DC/SVPWM /XYZ ==
  Ualph : Inport
  Ubata : Inport  Port=2
  T : Inport  Port=3
  Udc : Inport  Port=4
  Add : Sum
  Add1 : Sum  Inputs=+-
  Divide : Product  Inputs=**/
  Divide1 : Product  Inputs=**/
  Divide2 : Product  Inputs=**/
  Gain : Gain  Gain=sqrt(3)
  Gain1 : Gain  Gain=1/sqrt(3)
  Gain2 : Gain  Gain=3/2
  Gain3 : Gain  Gain=3/2
  Memory : Memory  InitialCondition=1
  X : Outport
  Y : Outport  Port=2
  Z : Outport  Port=3
  wires:
  Gain2/1 -> Y/1
  Gain3/1 -> Z/1
  Divide/1 -> X/1
  Divide2/1 -> Gain3/1
  Divide1/1 -> Gain2/1
  Udc/1 -> Memory/1
  T/1 -> Divide2/2, Divide/2, Divide1/2
  Add1/1 -> Divide2/1
  Add/1 -> Divide1/1
  Ualph/1 -> Add1/2, Add/2
  Gain1/1 -> Add1/1, Add/1
  Gain/1 -> Divide/1
  Ubata/1 -> Gain1/1, Gain/1
  Memory/1 -> Divide2/3, Divide1/3, Divide/3

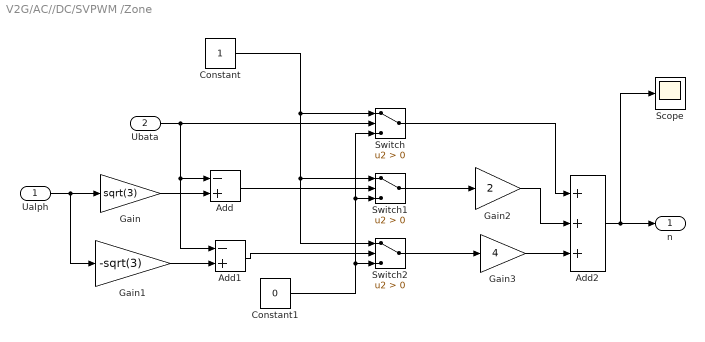
== system V2G/AC//DC/SVPWM /Zone ==
  Ualph : Inport
  Ubata : Inport  Port=2
  Add : Sum  Inputs=-+
  Add1 : Sum  Inputs=-+
  Add2 : Sum  Inputs=+++
  Constant : Constant
  Constant1 : Constant  Value=0
  Gain : Gain  Gain=sqrt(3)
  Gain1 : Gain  Gain=-sqrt(3)
  Gain2 : Gain  Gain=2
  Gain3 : Gain  Gain=4
  Scope : Scope
  Switch : Switch  Criteria=u2 > Threshold  SaturateOnIntegerOverflow=off  InputSameDT=off
  Switch1 : Switch  Criteria=u2 > Threshold  SaturateOnIntegerOverflow=off  InputSameDT=off
  Switch2 : Switch  Criteria=u2 > Threshold  SaturateOnIntegerOverflow=off  InputSameDT=off
  n : Outport
  wires:
  Add2/1 -> Scope/1, n/1
  Gain2/1 -> Add2/2
  Gain3/1 -> Add2/3
  Switch2/1 -> Gain3/1
  Switch1/1 -> Gain2/1
  Switch/1 -> Add2/1
  Add1/1 -> Switch2/2
  Add/1 -> Switch1/2
  Gain1/1 -> Add1/2
  Gain/1 -> Add/2
  Ualph/1 -> Gain/1, Gain1/1
  Ubata/1 -> Switch/2, Add1/1, Add/1
  Constant1/1 -> Switch2/3, Switch1/3, Switch/3
  Constant/1 -> Switch1/1, Switch2/1, Switch/1

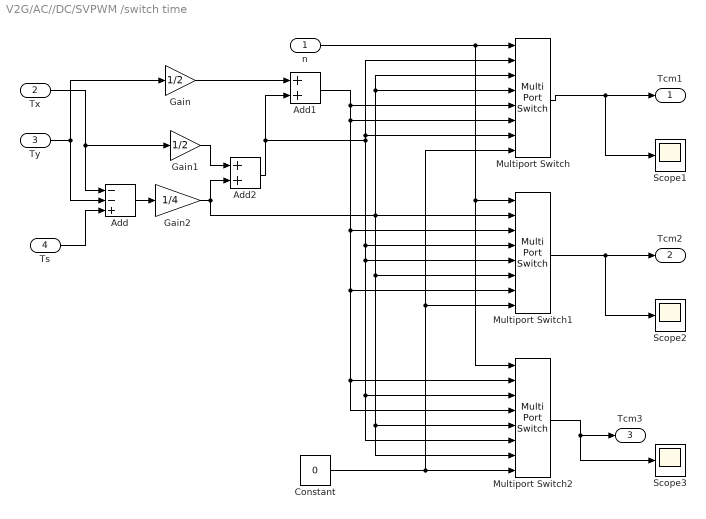
== system V2G/AC//DC/SVPWM /switch time ==
  n : Inport
  Tx : Inport  Port=2
  Ty : Inport  Port=3
  Ts : Inport  Port=4
  Add : Sum  Inputs=--+
  Add1 : Sum
  Add2 : Sum
  Constant : Constant  Value=0
  Gain : Gain  Gain=1/2
  Gain1 : Gain  Gain=1/2
  Gain2 : Gain  Gain=1/4
  Multiport Switch : MultiPortSwitch  Inputs=7  SaturateOnIntegerOverflow=off  InputSameDT=off
  Multiport Switch1 : MultiPortSwitch  Inputs=7  SaturateOnIntegerOverflow=off  InputSameDT=off
  Multiport Switch2 : MultiPortSwitch  Inputs=7  SaturateOnIntegerOverflow=off  InputSameDT=off
  Scope1 : Scope
  Scope2 : Scope
  Scope3 : Scope
  Tcm1 : Outport
  " Tcm2" : Outport  Port=2
  " Tcm3" : Outport  Port=3
  wires:
  Ty/1 -> Gain/1, Add/2
  Tx/1 -> Gain1/1, Add/1
  Add/1 -> Gain2/1
  Constant/1 -> Multiport Switch1/8, Multiport Switch/8, Multiport Switch2/8
  Add1/1 -> Multiport Switch/6, Multiport Switch1/7, Multiport Switch2/4, Multiport Switch2/2, Multiport Switch1/3, Multiport Switch/5
  n/1 -> Multiport Switch/1, Multiport Switch2/1, Multiport Switch1/1
  Gain/1 -> Add1/1
  Add2/1 -> Multiport Switch/7, Multiport Switch/2, Multiport Switch2/6, Multiport Switch2/3, Multiport Switch1/5, Multiport Switch1/4, Add1/2
  Gain2/1 -> Multiport Switch2/7, Multiport Switch2/5, Multiport Switch1/6, Multiport Switch/4, Multiport Switch/3, Multiport Switch1/2, Add2/2
  Gain1/1 -> Add2/1
  Multiport Switch2/1 -> Scope3/1, " Tcm3"/1
  Ts/1 -> Add/3
  Multiport Switch/1 -> Scope1/1, Tcm1/1
  Multiport Switch1/1 -> Scope2/1, " Tcm2"/1

== system V2G/DC//DC_Controller/Subsystem/PWM  ==
  D : Inport
  Add : Sum  Inputs=+-
  Constant3 : Constant
  Constant4 : Constant  Value=0
  Repeating Sequence1 : simulink/Sources/Repeating Sequence  rep_seq_t=[0 1e-4 2e-4]  rep_seq_y=[0 1 0]
  Scope : Scope
  Scope1 : Scope
  Switch : Switch  RndMeth=Round  ZeroCross=off  SaturateOnIntegerOverflow=off  InputSameDT=off
  PWM : Outport
  wires:
  Add/1 -> Switch/2
  Constant4/1 -> Switch/3
  Constant3/1 -> Switch/1
  Switch/1 -> Scope1/1, PWM/1
  D/1 -> Add/1
  Repeating Sequence1/1 -> Add/2, Scope/1

== system V2G/DC//DC_Controller/Subsystem1/Discrete PI Controller2 ==
  note: Discrete PID Controller
  note: Pierre Giroux, Gilbert Sybille
      | Power System Simulation Laboratory
      | IREQ, Hydro-Quebc
  Error : Inport
  Discrete-Time Integrator : DiscreteIntegrator  InitialCondition=Init  SampleTime=Ts  LimitOutput=on  UpperSaturationLimit=UpperLimit  LowerSaturationLimit=LowerLimit  ICPrevOutput=DiscIntNeverNeededParam  ICPrevScaledInput=DiscIntNeverNeededParam
  Kp4 : Gain  Gain=Kp  SaturateOnIntegerOverflow=on  OutDataTypeStr=Inherit: Same as input  ParamDataTypeStr=Inherit: Same as input
  Kp5 : Gain  Gain=Ki  SaturateOnIntegerOverflow=on  OutDataTypeStr=Inherit: Same as input  ParamDataTypeStr=Inherit: Same as input
  Saturation2 : Saturate  UpperLimit=UpperLimit  LowerLimit=LowerLimit
  Scope1 : Scope
  Scope7 : Scope
  Sum6 : Sum  InputSameDT=on  SaturateOnIntegerOverflow=on  OutDataTypeStr=Inherit: Same as first input
  Out : Outport  InitialOutput=0
  wires:
  Saturation2/1 -> Out/1
  Discrete-Time Integrator/1 -> Sum6/2, Scope1/1
  Kp4/1 -> Sum6/1, Scope7/1
  Kp5/1 -> Discrete-Time Integrator/1
  Sum6/1 -> Saturation2/1
  Error/1 -> Kp5/1, Kp4/1

== system V2G/DC//DC_Controller/Subsystem1/PWM  ==
  D : Inport
  Add : Sum  Inputs=+-
  Constant3 : Constant
  Constant4 : Constant  Value=0
  Logical Operator : Logic  Operator=NOT  AllPortsSameDT=off  OutDataTypeStr=boolean
  Repeating Sequence1 : simulink/Sources/Repeating Sequence  rep_seq_t=[0 1e-4 2e-4]  rep_seq_y=[0 1 0]
  Scope1 : Scope
  Switch : Switch  SaturateOnIntegerOverflow=off  InputSameDT=off
  PWM : Outport
  wires:
  Add/1 -> Switch/2
  Constant4/1 -> Switch/3
  Constant3/1 -> Switch/1
  D/1 -> Add/1
  Repeating Sequence1/1 -> Add/2
  Switch/1 -> Logical Operator/1
  Logical Operator/1 -> PWM/1, Scope1/1

== system V2G/AC//DC/Control Model/3 phase PLL double dq reframe user defined/+PARK+ ==
  alpha1 : Inport
  bata1 : Inport  Port=2
  angle : Inport  Port=3
  Fcn : Fcn  Expr=u(1)*cos(u(3))+u(2)*sin(u(3))
  Fcn1 : Fcn  Expr=-u(1)*sin(u(3))+u(2)*cos(u(3))
  Mux : Mux  Inputs=3
  Vd+ : Outport
  Vq+ : Outport  Port=2
  wires:
  alpha1/1 -> Mux/1
  bata1/1 -> Mux/2
  angle/1 -> Mux/3
  Mux/1 -> Fcn/1, Fcn1/1
  Fcn1/1 -> Vq+/1
  Fcn/1 -> Vd+/1

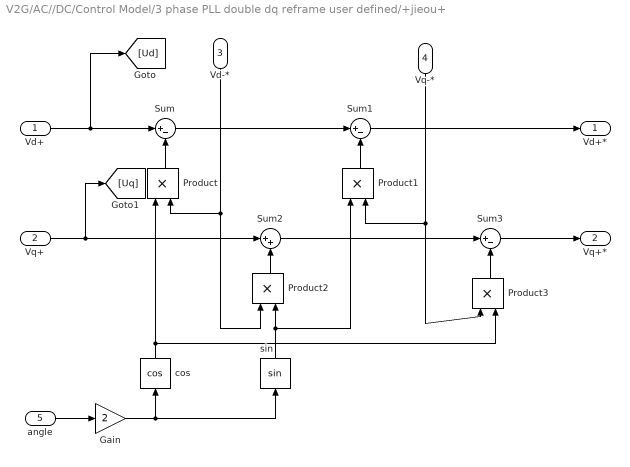
== system V2G/AC//DC/Control Model/3 phase PLL double dq reframe user defined/+jieou+ ==
  Vd+ : Inport
  Vq+ : Inport  Port=2
  Vd-* : Inport  Port=3
  Vq-* : Inport  Port=4
  angle : Inport  Port=5
  Gain : Gain  Gain=2
  Product{,1..3} (4 alike) : Product  RndMeth=Zero
  Sum : Sum  Inputs=|+-
  Sum1 : Sum  Inputs=|+-
  Sum2 : Sum  Inputs=|++
  Sum3 : Sum  Inputs=|+-
  cos : Trigonometry  Operator=cos
  sin : Trigonometry
  Vd+* : Outport
  Vq+* : Outport  Port=2
  wires:
  angle/1 -> Gain/1
  Gain/1 -> cos/1, sin/1
  sin/1 -> Product2/2, Product1/1
  Vd+/1 -> Sum/1, [Ud]
  cos/1 -> Product/1, Product3/2
  Vd-*/1 -> Product/2, Product2/1
  Product/1 -> Sum/2
  Vq+/1 -> Sum2/1, [Uq]
  Product2/1 -> Sum2/2
  Sum2/1 -> Sum3/1
  Vq-*/1 -> Product1/2, Product3/1
  Product3/1 -> Sum3/2
  Sum3/1 -> Vq+*/1
  Sum/1 -> Sum1/1
  Sum1/1 -> Vd+*/1
  Product1/1 -> Sum1/2

== system V2G/AC//DC/Control Model/3 phase PLL double dq reframe user defined/-PARK- ==
  alpha1 : Inport
  bata1 : Inport  Port=2
  angle : Inport  Port=3
  Fcn : Fcn  Expr=u(1)*cos(u(3))-u(2)*sin(u(3))
  Fcn1 : Fcn  Expr=u(1)*sin(u(3))+u(2)*cos(u(3))
  Mux : Mux  Inputs=3
  Vd- : Outport
  Vq- : Outport  Port=2
  wires:
  alpha1/1 -> Mux/1
  bata1/1 -> Mux/2
  angle/1 -> Mux/3
  Mux/1 -> Fcn/1, Fcn1/1
  Fcn1/1 -> Vq-/1
  Fcn/1 -> Vd-/1

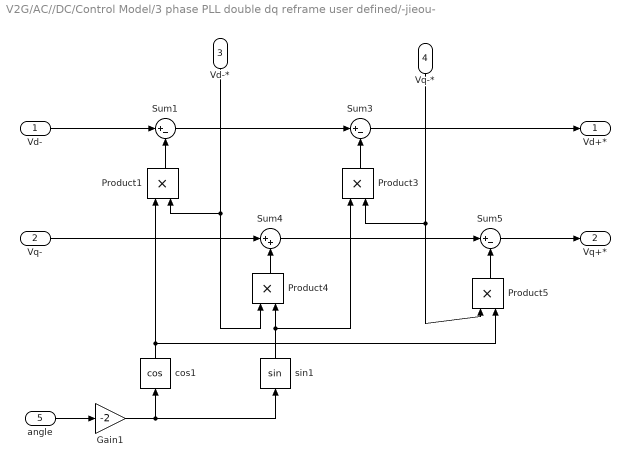
== system V2G/AC//DC/Control Model/3 phase PLL double dq reframe user defined/-jieou- ==
  Vd- : Inport
  Vq- : Inport  Port=2
  Vd-* : Inport  Port=3
  Vq-* : Inport  Port=4
  angle : Inport  Port=5
  Gain1 : Gain  Gain=-2
  Product{1,3..5} (4 alike) : Product  RndMeth=Zero
  Sum1 : Sum  Inputs=|+-
  Sum3 : Sum  Inputs=|+-
  Sum4 : Sum  Inputs=|++
  Sum5 : Sum  Inputs=|+-
  cos1 : Trigonometry  Operator=cos
  sin1 : Trigonometry
  Vd+* : Outport
  Vq+* : Outport  Port=2
  wires:
  angle/1 -> Gain1/1
  Gain1/1 -> cos1/1, sin1/1
  sin1/1 -> Product4/2, Product3/1
  Vd-/1 -> Sum1/1
  cos1/1 -> Product1/1, Product5/2
  Vd-*/1 -> Product1/2, Product4/1
  Product1/1 -> Sum1/2
  Vq-/1 -> Sum4/1
  Product4/1 -> Sum4/2
  Sum4/1 -> Sum5/1
  Vq-*/1 -> Product3/2, Product5/1
  Product5/1 -> Sum5/2
  Sum5/1 -> Vq+*/1
  Sum1/1 -> Sum3/1
  Sum3/1 -> Vd+*/1
  Product3/1 -> Sum3/2

== system V2G/AC//DC/Control Model/3 phase PLL double dq reframe user defined/CLARK ==
  Ua : Inport
  Ub : Inport  Port=2
  Uc : Inport  Port=3
  Fcn : Fcn  Expr=(2*u(1)-u(2)-u(3))/3
  Fcn1 : Fcn  Expr=(u(2)-u(3))*sqrt(3)/3
  Mux : Mux  Inputs=3
  alpha : Outport
  bata : Outport  Port=2
  wires:
  Ua/1 -> Mux/1
  Ub/1 -> Mux/2
  Uc/1 -> Mux/3
  Mux/1 -> Fcn/1, Fcn1/1
  Fcn/1 -> alpha/1
  Fcn1/1 -> bata/1
